simulink model "act1_simulink_sesion2"  (R2020a)
settings: Solver=ode1  StartTime=0.0  StopTime=10.0  FixedStep=0.001  RelTol=1e-3
values from neighbouring files (symbols this model uses):
  a_I = 1    [act1_script_sesion2.m]
  a_II = 10    [act1_script_sesion2.m]
  a_III = 100    [act1_script_sesion2.m]
  b_I = 1    [act1_script_sesion2.m]
  b_II = 10    [act1_script_sesion2.m]
  b_III = 100    [act1_script_sesion2.m]
settings Model: Creator=Jorjolo  LastModifiedBy=Jorjolo

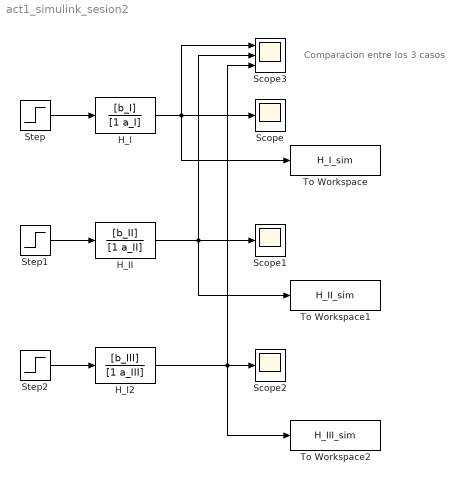
== system act1_simulink_sesion2 ==
  note: Comparacion entre los 3 casos
  H_I : TransferFcn  Numerator=[b_I]  Denominator=[1 a_I]
  H_I2 : TransferFcn  Numerator=[b_III]  Denominator=[1 a_III]
  H_II : TransferFcn  Numerator=[b_II]  Denominator=[1 a_II]
  Scope : Scope
  Scope1 : Scope
  Scope2 : Scope
  Scope3 : Scope  NumInputPorts=3
  Step : Step  SampleTime=0
  Step1 : Step  SampleTime=0
  Step2 : Step  SampleTime=0
  To Workspace : ToWorkspace  VariableName=H_I_sim  SaveFormat=Timeseries  SampleTime=-1
  To Workspace1 : ToWorkspace  VariableName=H_II_sim  SaveFormat=Timeseries  SampleTime=-1
  To Workspace2 : ToWorkspace  VariableName=H_III_sim  SaveFormat=Timeseries  SampleTime=-1
  wires:
  H_I2/1 -> To Workspace2/1, Scope3/3, Scope2/1
  H_II/1 -> To Workspace1/1, Scope3/2, Scope1/1
  Step/1 -> H_I/1
  Step1/1 -> H_II/1
  Step2/1 -> H_I2/1
  H_I/1 -> To Workspace/1, Scope3/1, Scope/1
